simulink library "angleBtwVecs_ul"  (R2020a)
settings: Solver=VariableStepAuto  StartTime=0.0  StopTime=10.0  RelTol=1e-3
libraries: vrlib x1
settings Model: Creator=Ayaz  LastModifiedBy=Ayaz

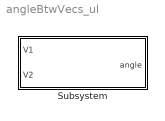
== system angleBtwVecs_ul ==
  Subsystem : Subsystem

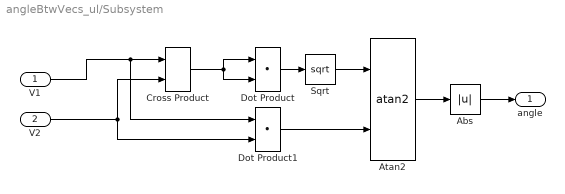
== system angleBtwVecs_ul/Subsystem ==
  V1 : Inport
  V2 : Inport  Port=2
  Abs : Abs
  Atan2 : Trigonometry  Operator=atan2
  Cross Product : vrlib/Utilities/Cross Product
  Dot Product : DotProduct  InputSameDT=on  OutDataTypeStr=Inherit: Inherit via internal rule
  Dot Product1 : DotProduct  InputSameDT=on  OutDataTypeStr=Inherit: Inherit via internal rule
  Sqrt : Sqrt  SaturateOnIntegerOverflow=on
  angle : Outport
  wires:
  V1/1 -> Dot Product1/1, Cross Product/1
  V2/1 -> Dot Product1/2, Cross Product/2
  Abs/1 -> angle/1
  Cross Product/1 -> Dot Product/1, Dot Product/2
  Dot Product/1 -> Sqrt/1
  Dot Product1/1 -> Atan2/2
  Atan2/1 -> Abs/1
  Sqrt/1 -> Atan2/1
